simulink model "inpguitest"  (Simulink 6.5)
settings: Solver=FixedStepDiscrete  StartTime=0.0  StopTime=inf  RelTol=1e-3
settings Model: Creator=nskandan  LastModifiedBy=nskandan

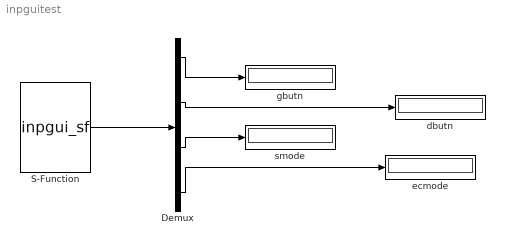
== system inpguitest ==
  Demux : Demux
  S-Function : S-Function  FunctionName=inpgui_sf  Parameters=0.005
  dbutn : Display
  ecmode : Display
  gbutn : Display
  smode : Display
  wires:
  S-Function/1 -> Demux/1
  Demux/1 -> gbutn/1
  Demux/2 -> dbutn/1
  Demux/3 -> smode/1
  Demux/4 -> ecmode/1
